simulink model "Project1_3_v2"  (R2024b)
settings: Solver=VariableStepAuto  StartTime=0.0  StopTime=100  RelTol=1e-3
model workspace (MAT data in the model file):
  J1 = 100
  J2 = 1
  T1 = 1
  b1 = 1
  b2 = 1
values from neighbouring files (symbols this model uses):
  A = 1    [Project1Part1Graphs.m]
  w_0 = 1    [Project1Part1Graphs.m]
settings Model: Creator=Ian  LastModifiedBy=Ian

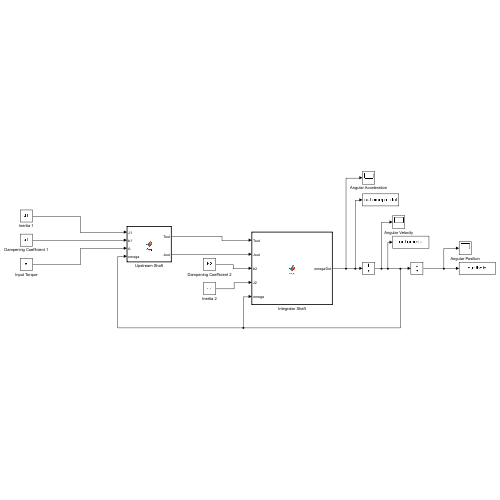
[thumbnail: Simulink's stored preview of the top-level diagram]
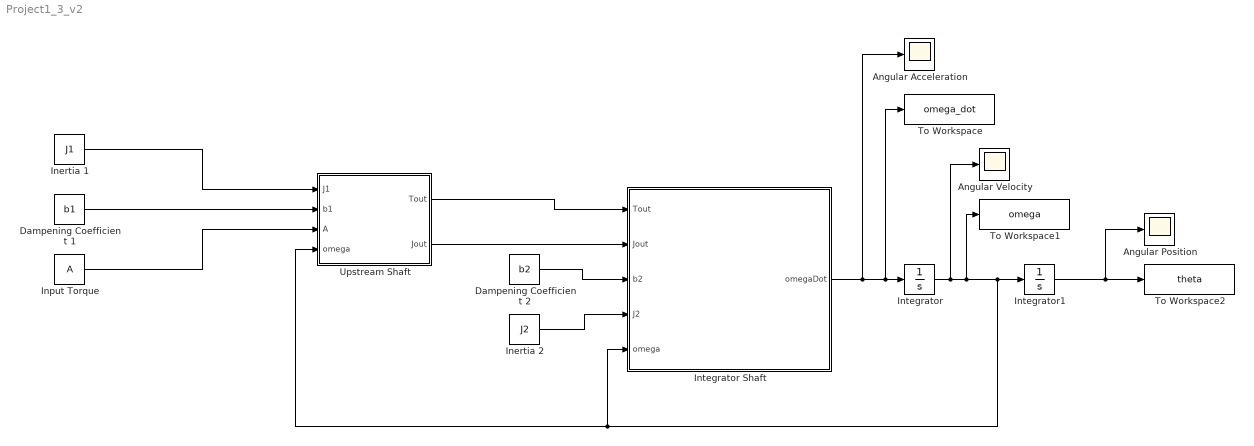
== system Project1_3_v2 ==
  Angular Acceleration : Scope
  Angular Position : Scope
  Angular Velocity : Scope
  Dampening Coefficient 1 : Constant  Value=b1
  Dampening Coefficient 2 : Constant  Value=b2
  Inertia 1 : Constant  Value=J1
  Inertia 2 : Constant  Value=J2
  Input Torque : Constant  Value=A
  Integrator : Integrator  InitialCondition=w_0
  Integrator Shaft : MATLAB Function  TreatAsAtomicUnit=on
  Integrator1 : Integrator
  To Workspace : ToWorkspace  VariableName=omega_dot  SaveFormat=Timeseries  SampleTime=-1
  To Workspace1 : ToWorkspace  VariableName=omega  SaveFormat=Timeseries  SampleTime=-1
  To Workspace2 : ToWorkspace  VariableName=theta  SaveFormat=Timeseries  SampleTime=-1
  Upstream Shaft : MATLAB Function  TreatAsAtomicUnit=on
  wires:
  Inertia 1/1 -> Upstream Shaft/1(J1)
  Dampening Coefficient 1/1 -> Upstream Shaft/2(b1)
  Input Torque/1 -> Upstream Shaft/3(A)
  Upstream Shaft/1(Tout) -> Integrator Shaft/1(Tout)
  Upstream Shaft/2(Jout) -> Integrator Shaft/2(Jout)
  Dampening Coefficient 2/1 -> Integrator Shaft/3(b2)
  Inertia 2/1 -> Integrator Shaft/4(J2)
  Integrator Shaft/1(omegaDot) -> Angular Acceleration/1, To Workspace/1, Integrator/1
  Integrator/1 -> Angular Velocity/1, To Workspace1/1, Upstream Shaft/4(omega), Integrator Shaft/5(omega), Integrator1/1
  Integrator1/1 -> Angular Position/1, To Workspace2/1

== matlab function Project1_3_v2/Integrator Shaft ==
  data: Tout input; omegaDot output; Jout input; b2 input; J2 input; omega input
function omegaDot = fcn(Tout, Jout, b2, J2, omega)

omegaDot = (Tout-(omega*b2))/(Jout+J2);

== matlab function Project1_3_v2/Upstream Shaft ==
  data: J1 input; Tout output; b1 input; A input; Jout output; omega input
function [Tout,Jout] = fcn(J1, b1, A, omega)

Tout = (omega*b1)+A;
Jout = J1;
